simulink model "W1P1"  (R2020b)
settings: Solver=VariableStepAuto  StartTime=0.0  StopTime=10.0  RelTol=1e-3
settings Model: Creator=saadh  LastModifiedBy=saadh

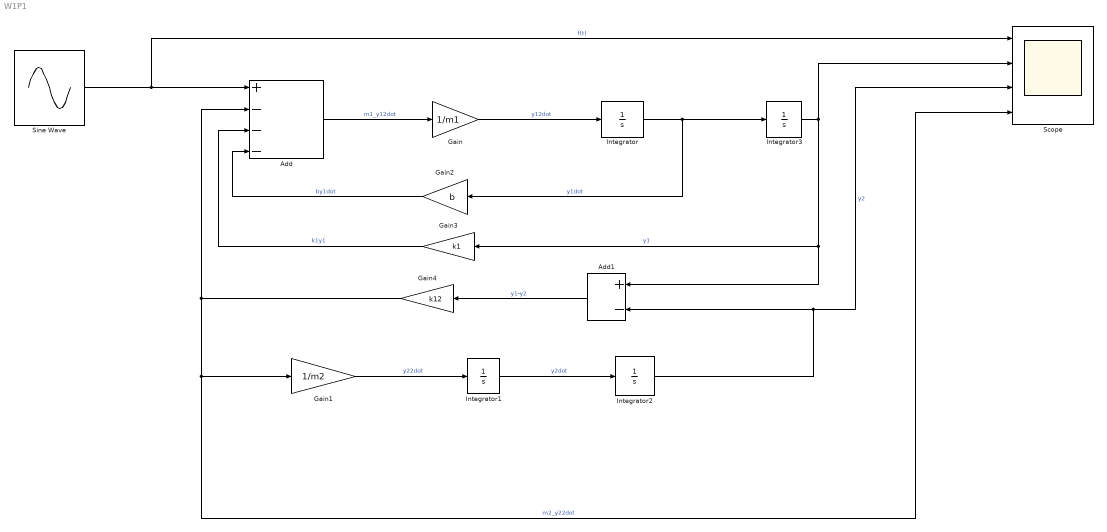
== system W1P1 ==
  Add : Sum  Inputs=+---
  Add1 : Sum  Inputs=+-
  Gain : Gain  Gain=1/m1  mask{m1=100}
  Gain1 : Gain  Gain=1/m2  mask{m2=80.0}
  Gain2 : Gain  Gain=b  mask{b=50}
  Gain3 : Gain  Gain=k1  mask{k1=50}
  Gain4 : Gain  Gain=k12  mask{k12=30.0}
  Integrator : Integrator  InitialCondition=1
  Integrator1 : Integrator
  Integrator2 : Integrator
  Integrator3 : Integrator
  Scope : Scope  NumInputPorts=4
  Sine Wave : Sin  Amplitude=2  Frequency=2*pi*10  SampleTime=0.005
  wires:
  Add/1 -> Gain/1  "m1_y12dot"
  Sine Wave/1 -> Scope/1, Add/1  "f(t)"
  Gain/1 -> Integrator/1  "y12dot"
  Integrator/1 -> Gain2/1, Integrator3/1  "y1dot"
  Gain2/1 -> Add/4  "by1dot"
  Integrator3/1 -> Scope/2, Gain3/1, Add1/1  "y1"
  Gain3/1 -> Add/3  "k1y1"
  Add1/1 -> Gain4/1  "y1-y2"
  Gain1/1 -> Integrator1/1  "y22dot"
  Integrator1/1 -> Integrator2/1  "y2dot"
  Integrator2/1 -> Scope/3, Add1/2  "y2"
  Gain4/1 -> Scope/4, Gain1/1, Add/2  "m2_y22dot"
